simulink model "sitl_atti"  (R2022b)
settings: Solver=FixedStepAuto  StartTime=0.0  StopTime=T  RelTol=1e-3
values from neighbouring files (symbols this model uses):
  b1 = 300    [eso.m]
  b2 = 30000    [eso.m]
  b3 = 1000000    [eso.m]
  dt = 1/500    (= 0.002)    [eso.m]    (also in sfhan.m = 0.005)
  h0 = u(3)    [sfhan.m]
undefined symbols (not defined in the file or in its folder): J, K, peak, r0xy, r0z, R_mea, w_mea
libraries: shared6dof x1, aerolibutil x1
settings Model: Creator=zzy  LastModifiedBy=zzy
settings DataIOCC: ReturnWorkspaceOutputs=off

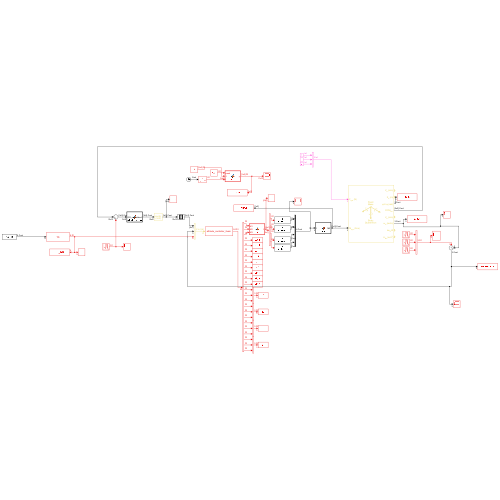
[thumbnail: Simulink's stored preview of the top-level diagram]
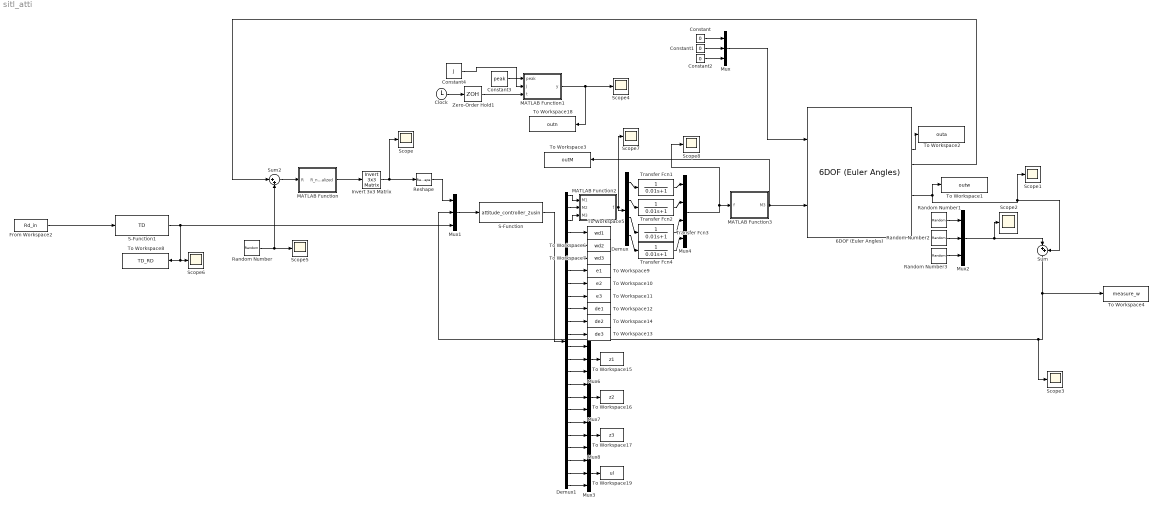
== system sitl_atti ==
  6DOF (Euler Angles) : shared6dof/6DOF (Euler Angles)  units=Metric (MKS)  mtype=Fixed  rep=Quaternion  xme_0=[0 0 0]  Vm_0=[0 0 0]  eul_0=[0 0 0]  pm_0=[0 0 0]  mass_0=m  mass_e=0.5  mass_f=2.0  inertia=J  inertia_e=eye(3)  inertia_f=2*eye(3)  k_quat=1.0  vre_flag=on  abi_flag=off  aMode=0  xme_statename=''  Vm_statename=''  eul_statename=''  quat_statename=''  pm_statename=''  mass_statename=''
  Clock : Clock
  Constant : Constant  Value=0
  Constant1 : Constant  Value=0
  Constant2 : Constant  Value=0
  Constant3 : Constant  Value=peak  SampleTime=dt
  Constant4 : Constant  Value=J  SampleTime=dt
  Demux : Demux
  Demux1 : Demux  Outputs=24
  From Workspace2 : FromWorkspace  VariableName=Rd_in
  Invert 3x3 Matrix : aerolibutil/Invert  3x3 Matrix
  MATLAB Function : MATLAB Function  TreatAsAtomicUnit=on
  MATLAB Function1 : MATLAB Function  TreatAsAtomicUnit=on
  MATLAB Function2 : MATLAB Function  TreatAsAtomicUnit=on
  MATLAB Function3 : MATLAB Function  TreatAsAtomicUnit=on
  Mux{,1..3,6..8} (7 alike) : Mux  Inputs=3
  Mux4 : Mux
  Random Number : RandomNumber  Variance=R_mea  SampleTime=dt
  Random Number1 : RandomNumber  Variance=w_mea  SampleTime=dt
  Random Number2 : RandomNumber  Variance=w_mea  Seed=78237  SampleTime=dt
  Random Number3 : RandomNumber  Variance=w_mea  Seed=456  SampleTime=dt
  Reshape : Reshape  OutputDimensionality=Column vector (2-D)
  S-Function : S-Function  FunctionName=attitude_controller_2usin  Parameters=dt,J,K,b1,b2,b3  SFunctionDeploymentMode=off  EnableBusSupport=off
  S-Function1 : S-Function  FunctionName=TD  Parameters=dt,r0xy,r0z,h0  SFunctionDeploymentMode=off  EnableBusSupport=off
  Scope{,1..8} (9 alike) : Scope
  Sum : Sum  Inputs=|++
  Sum2 : Sum  Inputs=|++
  To Workspace1 : ToWorkspace  VariableName=outw  SampleTime=-1
      settings: Save2DSignal=2-D array (concatenate along first dimension)
  To Workspace10 : ToWorkspace  VariableName=e2  SampleTime=-1
      settings: Save2DSignal=2-D array (concatenate along first dimension)
  To Workspace11 : ToWorkspace  VariableName=e3  SampleTime=-1
      settings: Save2DSignal=2-D array (concatenate along first dimension)
  To Workspace12 : ToWorkspace  VariableName=de1  SampleTime=-1
      settings: Save2DSignal=2-D array (concatenate along first dimension)
  To Workspace13 : ToWorkspace  VariableName=de3  SampleTime=-1
      settings: Save2DSignal=2-D array (concatenate along first dimension)
  To Workspace14 : ToWorkspace  VariableName=de2  SampleTime=-1
      settings: Save2DSignal=2-D array (concatenate along first dimension)
  To Workspace15 : ToWorkspace  VariableName=z1  SampleTime=-1
      settings: Save2DSignal=2-D array (concatenate along first dimension)
  To Workspace16 : ToWorkspace  VariableName=z2  SampleTime=-1
      settings: Save2DSignal=2-D array (concatenate along first dimension)
  To Workspace17 : ToWorkspace  VariableName=z3  SampleTime=-1
      settings: Save2DSignal=2-D array (concatenate along first dimension)
  To Workspace18 : ToWorkspace  VariableName=outn  SampleTime=-1
      settings: Save2DSignal=2-D array (concatenate along first dimension)
  To Workspace19 : ToWorkspace  VariableName=ul  SampleTime=-1
      settings: Save2DSignal=2-D array (concatenate along first dimension)
  To Workspace2 : ToWorkspace  VariableName=outa  SampleTime=-1
      settings: Save2DSignal=2-D array (concatenate along first dimension)
  To Workspace3 : ToWorkspace  VariableName=outM  SampleTime=-1
      settings: Save2DSignal=2-D array (concatenate along first dimension)
  To Workspace4 : ToWorkspace  VariableName=measure_w  SampleTime=-1
      settings: Save2DSignal=2-D array (concatenate along first dimension)
  To Workspace5 : ToWorkspace  VariableName=wd1  SampleTime=-1
      settings: Save2DSignal=2-D array (concatenate along first dimension)
  To Workspace6 : ToWorkspace  VariableName=wd2  SampleTime=-1
      settings: Save2DSignal=2-D array (concatenate along first dimension)
  To Workspace7 : ToWorkspace  VariableName=wd3  SampleTime=-1
      settings: Save2DSignal=2-D array (concatenate along first dimension)
  To Workspace8 : ToWorkspace  VariableName=TD_RD  SampleTime=-1
      settings: Save2DSignal=2-D array (concatenate along first dimension)
  To Workspace9 : ToWorkspace  VariableName=e1  SampleTime=-1
      settings: Save2DSignal=2-D array (concatenate along first dimension)
  Transfer Fcn{1..4} (4 alike) : TransferFcn  Denominator=[0.01 1]
  Zero-Order Hold1 : ZeroOrderHold  SampleTime=-1
  wires:
  Constant1/1 -> Mux/2
  Constant/1 -> Mux/1
  Constant2/1 -> Mux/3
  Mux/1 -> 6DOF (Euler Angles)/1
  6DOF (Euler Angles)/6 -> Sum/2, Scope1/1, To Workspace1/1
  Invert 3x3 Matrix/1 -> Reshape/1, Scope/1
  Mux1/1 -> S-Function/1
  Reshape/1 -> Mux1/1
  6DOF (Euler Angles)/3 -> To Workspace2/1
  Sum/1 -> Mux1/2, Scope3/1, To Workspace4/1
  Random Number1/1 -> Mux2/1
  Random Number2/1 -> Mux2/2
  Random Number3/1 -> Mux2/3
  Mux2/1 -> Scope2/1, Sum/1
  Transfer Fcn1/1 -> Mux4/1
  Demux/1 -> Transfer Fcn1/1
  Random Number/1 -> Sum2/2, Scope5/1
  6DOF (Euler Angles)/4 -> Sum2/1
  Sum2/1 -> MATLAB Function/1(R)
  MATLAB Function/1(R_normalized) -> Invert 3x3 Matrix/1
  S-Function/1 -> Demux1/1
  Demux1/1 -> MATLAB Function2/1(M1)
  Demux1/2 -> MATLAB Function2/2(M2)
  Demux1/3 -> MATLAB Function2/3(M3)
  Demux1/4 -> To Workspace5/1
  Demux1/5 -> To Workspace6/1
  Demux1/6 -> To Workspace7/1
  S-Function1/1 -> To Workspace8/1, Scope6/1, Mux1/3
  Demux1/7 -> To Workspace9/1
  Demux1/8 -> To Workspace10/1
  Demux1/9 -> To Workspace11/1
  Demux1/10 -> To Workspace12/1
  Demux1/11 -> To Workspace14/1
  Demux1/12 -> To Workspace13/1
  From Workspace2/1 -> S-Function1/1
  Demux1/13 -> Mux6/1
  Demux1/14 -> Mux6/2
  Demux1/15 -> Mux6/3
  Mux6/1 -> To Workspace15/1
  Demux1/18 -> Mux7/3
  Demux1/16 -> Mux7/1
  Demux1/17 -> Mux7/2
  Mux7/1 -> To Workspace16/1
  Demux1/21 -> Mux8/3
  Demux1/19 -> Mux8/1
  Demux1/20 -> Mux8/2
  Mux8/1 -> To Workspace17/1
  Constant3/1 -> MATLAB Function1/1(peak)
  Clock/1 -> Zero-Order Hold1/1
  MATLAB Function1/1(y) -> To Workspace18/1, Scope4/1
  Zero-Order Hold1/1 -> MATLAB Function1/3(t)
  Constant4/1 -> MATLAB Function1/2(J)
  Mux3/1 -> To Workspace19/1
  Demux1/22 -> Mux3/1
  Demux1/23 -> Mux3/2
  Demux1/24 -> Mux3/3
  MATLAB Function2/1(f) -> Demux/1, Scope7/1
  Transfer Fcn2/1 -> Mux4/2
  Demux/2 -> Transfer Fcn2/1
  Transfer Fcn3/1 -> Mux4/3
  Demux/3 -> Transfer Fcn3/1
  Transfer Fcn4/1 -> Mux4/4
  Demux/4 -> Transfer Fcn4/1
  MATLAB Function3/1(M3) -> To Workspace3/1, 6DOF (Euler Angles)/2
  Mux4/1 -> Scope8/1, MATLAB Function3/1(f)

== matlab function sitl_atti/MATLAB Function ==
  data: R input; R_normalized output
function R_normalized = normalizeRotationMatrix(R)
% Normalize a rotation matrix using SVD
    [U, ~, V] = svd(R);
    R_normalized = U * V';
end

== matlab function sitl_atti/MATLAB Function2 ==
  data: M1 input; M2 input; f output; M3 input
function f = fcn(M1,M2,M3)
d1=0.073*2;
d2=0.085*2;
ctf=0.01;
A=[   -d1/2 d1/2 d1/2 -d1/2;
   d2/2 -d2/2 d2/2 -d2/2;
   ctf ctf -ctf -ctf;
   1 1 1 1;];
f = inv(A)*[M1;M2;M3;6.25];

end

== matlab function sitl_atti/MATLAB Function3 ==
  data: f input; M3 output
function M3 = fcn(f)
d1=0.073*2;
d2=0.085*2;
ctf=0.01;
A=[   -d1/2 d1/2 d1/2 -d1/2;
   d2/2 -d2/2 d2/2 -d2/2;
   ctf ctf -ctf -ctf;
   1 1 1 1;];
M = A*f;
M3 =M(1:3)';
end

== matlab function sitl_atti/MATLAB Function1 ==
  data: peak input; J input; y output; t input
function y = fcn(peak,J,t)
white_noise = peak * randn([1,3]);
% [b, a] = butter(1, 10 / (200 / 2));  % 低通滤波器设计
% y = filter(b, a, white_noise);

m1= sign(sin(0.9*t)) + cos(0.9*t);
m2 = sign(sin(0.9*t)) + cos(0.3*t);
m3 = 0.3*sin(0.3*t);
% m1=0;
% m3=0
% m2=sin(t);
y=(white_noise+[m1,m2,m3])*J*0;
end
